simulink model "SpiderHalfCentre_SingleLeg"  (R2022b)
settings: Solver=ode4  StartTime=0.0  StopTime=30  FixedStep=1e-3  RelTol=1e-3
undefined symbols (not defined in the file): t1, t2, Vus0
libraries: vexv5lib x4, vexcommonlib x2, Vex_V5_Simulink_Expansion x2
settings Model: Creator=Serious Chimp  LastModifiedBy=Serious Chimp
settings SolverCC: EnableFixedStepZeroCrossing=on
settings OptimizationCC: EnhancedBackFolding=on  PassReuseOutputArgsAs=Individual arguments  ZeroExternalMemoryAtStartup=off  ZeroInternalMemoryAtStartup=off  MaxStackSize=64  OptimizeBlockOrder=speed  DifferentSizesBufferReuse=on  OptimizationCustomize=off  EfficientTunableParamExpr=on
settings DebuggingCC: ParameterTunabilityLossMsg=error
settings HardwareCC: ProdBitPerPointer=32  ProdBitPerSizeT=32  ProdBitPerPtrDiffT=32  ProdLargestAtomicInteger=Long  ProdLargestAtomicFloat=Double  ProdWordSize=32  ProdHWDeviceType=ARM Compatible->ARM Cortex  UseEmbeddedCoderFeatures=off
settings SFSimCC: MATLABDynamicMemAlloc=off
settings RTWCC: Description=Embedded Coder  SystemTargetFile=ert.tlc  HardwareBoard=VEX V5 Robot Brain  TLCOptions="-aInlineSetEventsForThisBaseRateFcn=TLC_FALSE -aSuppressMultiTaskScheduler=TLC_FALSE  -aRateBasedStepFcn=0"  TemplateMakefile=ert_default_tmf  Toolchain=GNU Tools for ARM Embedded Processors
settings CodeAppCC: ForceParamTrailComments=on  IgnoreCustomStorageClasses=off  OperatorAnnotations=on  SimulinkDataObjDesc=on  SFDataObjDesc=on  InsertBlockDesc=on
settings ERTTargetCC: SupportNonInlinedSFcns=on  ExtModeTransport=3  ExtModeStaticAlloc=on  ExtModeStaticAllocSize=2048  ExtModeMexFile=ext_xcp  ExtModeIntrfLevel=Level2 - Open

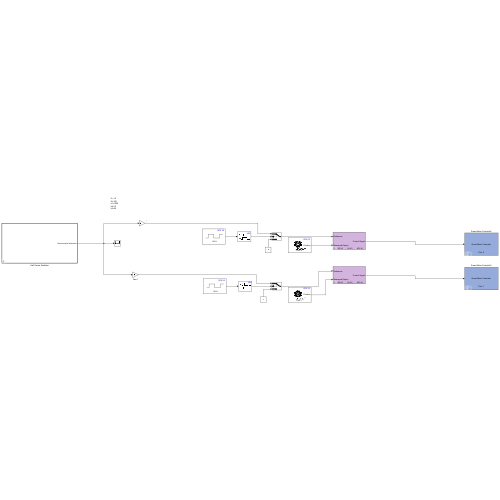
[thumbnail: Simulink's stored preview of the top-level diagram]
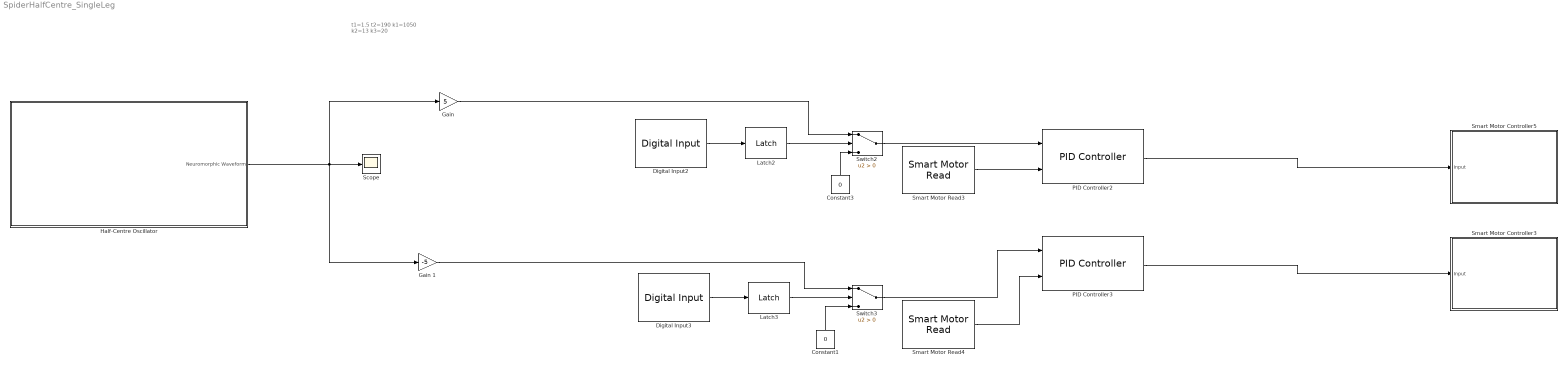
== system SpiderHalfCentre_SingleLeg ==
  note: t1=1.5
      | t2=190
      | k1=1050
      | k2=13
      | k3=20
  Constant1 : Constant  Value=0
  Constant3 : Constant  Value=0
  Digital Input2 : vexv5lib/Sensors/Digital Input  smartPort3wire=None  port=H  SampleTime=0.2
  Digital Input3 : vexv5lib/Sensors/Digital Input  smartPort3wire=None  port=H  SampleTime=0.2
  Gain : Gain  Gain=5
  Gain 1 : Gain  Gain=-5
  Half-Centre Oscillator : Subsystem  TreatAsAtomicUnit=on  mask{tau_s_A=t1, tau_us_A=t2, GB_A=-20, tau_s_B=t1, tau_us_B=t2, GB_B=-20, pain_threshold=2, pain_intensity=2, delay=0}
      mask prompts: tau_s_A "A - tau_s"; tau_us_A "A - tau_us"; GB_A "A - Inhibitory Synapse Threshold, GB_A"; tau_s_B "B - tau_s"; tau_us_B "B - tau_us"; GB_B "B - Inhibitory Synapse Threshold, GB_B"; pain_threshold "Range of Motion Position Threshold, pain_threshold"; pain_intensity "Range of Motion Intensity, pain_intensity"
  Latch2 : vexcommonlib/Latch  output0=off  BlockPlatform=vexv5
      settings: LibrarySourceBlock=vexv5lib/Utilities/Latch
  Latch3 : vexcommonlib/Latch  output0=off  BlockPlatform=vexv5
      settings: LibrarySourceBlock=vexv5lib/Utilities/Latch
  PID Controller2 : Vex_V5_Simulink_Expansion/Core Blocks/PID Controller  KP=k1  KI=k3  KD=k2  LimitOutput=off  limitHigh=0  limitLow=0  AntiWindupMode=none  kb=0
  PID Controller3 : Vex_V5_Simulink_Expansion/Core Blocks/PID Controller  KP=k1  KI=k3  KD=k2  LimitOutput=off  limitHigh=0  limitLow=0  AntiWindupMode=none  kb=0
  Scope : Scope
  Smart Motor Controller3 : Subsystem  AncestorBlock=Vex_V5_Simulink_Expansion/Core Blocks/Smart Motor Controller  mask(Smart Motor Controller){motorPort=1, OperationMode=Advanced Control, MotorBrakeMode=Coast}
      mask prompts: motorPort "Smart Port:"; OperationMode "Control Mode:"; MotorBrakeMode "Braking Mode:"
      mask help: Controls the Vex Smart Motor via the chosen method.
      mask TypeOptions motorPort: Advanced_SmartMotorWrite/motorPort
      mask TypeOptions OperationMode: Advanced_SmartMotorWrite/OperationMode
      mask TypeOptions MotorBrakeMode: Advanced_SmartMotorWrite/MotorBrakeMode
      mask DialogControl Container3 Prompt: Smart Motor Configuration
      mask Display:
      | %mode = get_param(gcb, 'control');
      | port = get_param(gcb, 'motorPort');
      | %text(0.3,0.45,[mode]);
      | 
      | text(0.5,0.5, 'Smart Motor Controller','HorizontalAlignment','center');
      | text(0.42,0.15, ['Port: ',port]);
  Smart Motor Controller5 : Subsystem  AncestorBlock=Vex_V5_Simulink_Expansion/Core Blocks/Smart Motor Controller  mask(Smart Motor Controller){motorPort=2, OperationMode=Advanced Control, MotorBrakeMode=Coast}
      mask prompts: motorPort "Smart Port:"; OperationMode "Control Mode:"; MotorBrakeMode "Braking Mode:"
      mask help: Controls the Vex Smart Motor via the chosen method.
      mask TypeOptions motorPort: Advanced_SmartMotorWrite/motorPort
      mask TypeOptions OperationMode: Advanced_SmartMotorWrite/OperationMode
      mask TypeOptions MotorBrakeMode: Advanced_SmartMotorWrite/MotorBrakeMode
      mask DialogControl Container3 Prompt: Smart Motor Configuration
      mask Display:
      | %mode = get_param(gcb, 'control');
      | port = get_param(gcb, 'motorPort');
      | %text(0.3,0.45,[mode]);
      | 
      | text(0.5,0.5, 'Smart Motor Controller','HorizontalAlignment','center');
      | text(0.42,0.15, ['Port: ',port]);
  Smart Motor Read3 : vexv5lib/Sensors/Smart Motor Read  motorPort=2  EncoderUnit=Degrees  resetOption=No reset  additionalOutput=off  SampleTime=0.01
  Smart Motor Read4 : vexv5lib/Sensors/Smart Motor Read  motorPort=1  EncoderUnit=Degrees  resetOption=No reset  additionalOutput=off  SampleTime=0.01
  Switch2 : Switch  Criteria=u2 > Threshold  SaturateOnIntegerOverflow=off  InputSameDT=off
  Switch3 : Switch  Criteria=u2 > Threshold  SaturateOnIntegerOverflow=off  InputSameDT=off
  wires:
  Smart Motor Read3/1 -> PID Controller2/2
  PID Controller2/1 -> Smart Motor Controller5/1(" Input")
  Gain 1/1 -> Switch3/1
  Digital Input2/1 -> Latch2/1
  Smart Motor Read4/1 -> PID Controller3/2
  Switch3/1 -> PID Controller3/1
  Constant3/1 -> Switch2/3
  Constant1/1 -> Switch3/3
  PID Controller3/1 -> Smart Motor Controller3/1(" Input")
  Gain/1 -> Switch2/1
  Latch3/1 -> Switch3/2
  Switch2/1 -> PID Controller2/1
  Digital Input3/1 -> Latch3/1
  Latch2/1 -> Switch2/2
  Half-Centre Oscillator/1(Neuromorphic Waveform) -> Scope/1, Gain/1, Gain 1/1

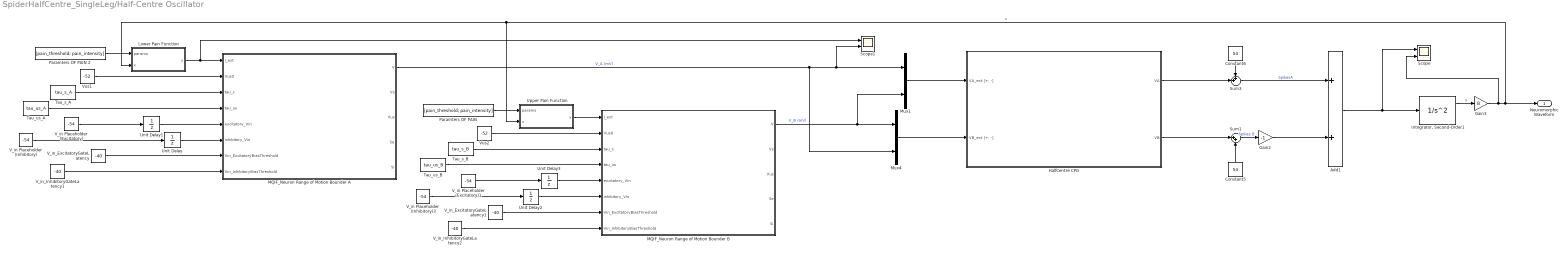
== system SpiderHalfCentre_SingleLeg/Half-Centre Oscillator ==
  Add1 : Sum
  Constant5 : Constant  Value=54
  Constant6 : Constant  Value=54
  Gain2 : Gain  Gain=-1
  Gain3 : Gain  Gain=8
  HalfCentre CPG : Subsystem  TreatAsAtomicUnit=on  mask{tau_s_A=t1, tau_us_A=t2, gSyn_excitatory_A=0.5, gSyn_inhibitory_A=0.5, tauSyn_excitatory_A=50, tauSyn_inhibitory_A=50, GB_A=-20, tau_s_B=t1, tau_us_B=t2, gSyn_excitatory_B=0.5, gSyn_inhibitory_B=0.5, tauSyn_excitatory_B=50, tauSyn_inhibitory_B=50, GB_B=-15, GB_excitatory=-40}
      mask prompts: tau_s_A "A - tau_s"; tau_us_A "A - tau_us"; gSyn_excitatory_A "A - Excitatory Synaptic Conductance, gSyn_excitatory"; gSyn_inhibitory_A "A - Inhibitory Synaptic Conductance, gSyn_inhibitory"; tauSyn_excitatory_A "A - Excitatory Synaptic Time Constant, tauSyn_excitatory"; tauSyn_inhibitory_A "A - Inhibitory Synaptic Time Constant, tauSyn_inhibitory"; GB_A "A - Inhibitory Synapse Threshold, GB_A"; tau_s_B "B - tau_s"; tau_us_B "B - tau_us"; gSyn_excitatory_B "B - Excitatory Synaptic Conductance, gSyn_excitatory"; gSyn_inhibitory_B "B - Inhibitory Synaptic Conductance, gSyn_inhibitory"; tauSyn_excitatory_B "B - Excitatory Synaptic Time Constant, tauSyn_excitatory"; tauSyn_inhibitory_B "B - Inhibitory Synaptic Time Constant, tauSyn_inhibitory"; GB_B "B - Inhibitory Synapse Threshold, GB_B"; GB_excitatory "Excitatory Gate Biases, GB_excitatory"
      mask Display: image('$imagefile'); % Use "Edit Image" on toolstrip to change.
  "Integrator, Second-Order1" : SecondOrderIntegrator
  Lower Pain Function : MATLAB Function  TreatAsAtomicUnit=on
  MQIF_Neuron Range of Motion Bounder A : Subsystem  TreatAsAtomicUnit=on  mask{V0=-52, Vs0=-50, V_threshold=20, V_reset=-45, Vs_reset=7.5, delta_Vus=1.7, g_f=1.0, g_s=0.5, g_us=0.015, C=0.82, Ve_syn=0, Vi_syn=-80, g_syn_excitatory=45, g_syn_inhibitory=45, tauSyn_excitatory=7, tauSyn_inhibitory=7, k=250}
      mask prompts: V0 "Equilibrium V0"; Vs0 "Equilibrium Vs0"; V_threshold "Threshold for Spike, V_thresh"; V_reset "After-spike Reset Votlage, V_r"; Vs_reset "After-spike Reset Vs, Vs_r"; delta_Vus "Vus After-spike Memory, delta_Vus"; g_f "I Conductance, g_f"; g_s "I_us Conductance, g_s"; g_us "I_us Conductance, g_us"; C "Capacitance, C"; Ve_syn "Equilibrium Inhibitory Synapse Voltage, Ve_syn"; Vi_syn "Equilibrium Inhibitory Synapse Voltage, Vi_syn"; g_syn_excitatory "Excitatory Synapse Conductance, g_syn_excitatory"; g_syn_inhibitory "Inhibitory Synapse Conductance, g_syn_inhibitory"; tauSyn_excitatory "Excitatory Synapse Time Constant, tauSyn_excitatory"; tauSyn_inhibitory "Inhibitory Synapse Time Constant, tauSyn_inhibitory"; k "Speed/Rate Constant, k"
      mask DialogControl NeuronStateVariables Prompt: Parameters
  MQIF_Neuron Range of Motion Bounder B : Subsystem  TreatAsAtomicUnit=on  mask{V0=-52, Vs0=-50, V_threshold=20, V_reset=-45, Vs_reset=7.5, delta_Vus=1.7, g_f=1.0, g_s=0.5, g_us=0.015, C=0.82, Ve_syn=0, Vi_syn=-80, g_syn_excitatory=45, g_syn_inhibitory=45, tauSyn_excitatory=7, tauSyn_inhibitory=7, k=250}
      mask prompts: V0 "Equilibrium V0"; Vs0 "Equilibrium Vs0"; V_threshold "Threshold for Spike, V_thresh"; V_reset "After-spike Reset Votlage, V_r"; Vs_reset "After-spike Reset Vs, Vs_r"; delta_Vus "Vus After-spike Memory, delta_Vus"; g_f "I Conductance, g_f"; g_s "I_us Conductance, g_s"; g_us "I_us Conductance, g_us"; C "Capacitance, C"; Ve_syn "Equilibrium Inhibitory Synapse Voltage, Ve_syn"; Vi_syn "Equilibrium Inhibitory Synapse Voltage, Vi_syn"; g_syn_excitatory "Excitatory Synapse Conductance, g_syn_excitatory"; g_syn_inhibitory "Inhibitory Synapse Conductance, g_syn_inhibitory"; tauSyn_excitatory "Excitatory Synapse Time Constant, tauSyn_excitatory"; tauSyn_inhibitory "Inhibitory Synapse Time Constant, tauSyn_inhibitory"; k "Speed/Rate Constant, k"
      mask DialogControl NeuronStateVariables Prompt: Parameters
  Mux1 : Mux  Inputs=2
  Mux4 : Mux  Inputs=2
  Paramters OF PAIN : Constant  Value=[pain_threshold; pain_intensity]
  Paramters OF PAIN 2 : Constant  Value=[pain_threshold; pain_intensity]
  Scope : Scope  NumInputPorts=2
  Scope1 : Scope  NumInputPorts=2
  Sum1 : Sum  Inputs=|++
  Sum3 : Sum  Inputs=++|
  Tau_s_A : Constant  Value=tau_s_A
  Tau_s_B : Constant  Value=tau_s_B
  Tau_us_A : Constant  Value=tau_us_A
  Tau_us_B : Constant  Value=tau_us_B
  Unit Delay{,1..3} (4 alike) : UnitDelay  InitialCondition=-54  SampleTime=-1  HasFrameUpgradeWarning=on
  Upper Pain Function : MATLAB Function  TreatAsAtomicUnit=on
  V_in Placeholder (Excitatory) : Constant  Value=-54
  V_in Placeholder (Excitatory)1 : Constant  Value=-54
  V_in Placeholder (Inhibitory) : Constant  Value=-54
  V_in Placeholder (Inhibitory)3 : Constant  Value=-54
  V_in_ExcitatoryGateLatency : Constant  Value=-40
  V_in_ExcitatoryGateLatency1 : Constant  Value=-40
  V_in_InhibitoryGateLatency1 : Constant  Value=-40
  V_in_InhibitoryGateLatency2 : Constant  Value=-40
  Vus1 : Constant  Value=-52
  Vus2 : Constant  Value=-52
  Neuromorphic Waveform : Outport
  wires:
  Constant5/1 -> Sum1/2
  MQIF_Neuron Range of Motion Bounder B/1(V) -> Mux1/2, Mux4/1  "V_B (mV)"
  V_in_ExcitatoryGateLatency/1 -> MQIF_Neuron Range of Motion Bounder A/7(Vin_ExcitatoryBiasThreshold)
  V_in Placeholder (Inhibitory)3/1 -> Unit Delay2/1
  Gain2/1 -> Add1/2
  V_in_InhibitoryGateLatency2/1 -> MQIF_Neuron Range of Motion Bounder B/8(Vin_InhibitoryBiasThreshold)
  Vus1/1 -> MQIF_Neuron Range of Motion Bounder A/2(Vus0)
  V_in Placeholder (Excitatory)/1 -> Unit Delay1/1
  Mux4/1 -> HalfCentre CPG/2(VB_ext [+; -])
  Unit Delay2/1 -> MQIF_Neuron Range of Motion Bounder B/6(inhibitory_Vin)
  Unit Delay/1 -> MQIF_Neuron Range of Motion Bounder A/6(inhibitory_Vin)
  Tau_s_B/1 -> MQIF_Neuron Range of Motion Bounder B/3(tau_s)
  Vus2/1 -> MQIF_Neuron Range of Motion Bounder B/2(Vus0)
  V_in Placeholder (Inhibitory)/1 -> Unit Delay/1
  "Integrator, Second-Order1"/1 -> Gain3/1  "x"
  V_in_ExcitatoryGateLatency1/1 -> MQIF_Neuron Range of Motion Bounder B/7(Vin_ExcitatoryBiasThreshold)
  Gain3/1 -> Scope/2, Neuromorphic Waveform/1, Upper Pain Function/2(x), Lower Pain Function/2(x)  "x"
  Sum3/1 -> Add1/1  "SpikesA"
  HalfCentre CPG/1(VA) -> Sum3/2
  V_in Placeholder (Excitatory)1/1 -> Unit Delay3/1
  Tau_us_A/1 -> MQIF_Neuron Range of Motion Bounder A/4(tau_us)
  Add1/1 -> Scope/1, "Integrator, Second-Order1"/1
  V_in_InhibitoryGateLatency1/1 -> MQIF_Neuron Range of Motion Bounder A/8(Vin_InhibitoryBiasThreshold)
  Unit Delay1/1 -> MQIF_Neuron Range of Motion Bounder A/5(excitatory_Vin)
  MQIF_Neuron Range of Motion Bounder A/1(V) -> Mux4/2, Scope1/2, Mux1/1  "V_A (mV)"
  Tau_s_A/1 -> MQIF_Neuron Range of Motion Bounder A/3(tau_s)
  Lower Pain Function/1(y) -> Scope1/1, MQIF_Neuron Range of Motion Bounder A/1(I_ext)
  Tau_us_B/1 -> MQIF_Neuron Range of Motion Bounder B/4(tau_us)
  Mux1/1 -> HalfCentre CPG/1(VA_ext [+; -])
  HalfCentre CPG/2(VB) -> Sum1/1
  Sum1/1 -> Gain2/1  "Spikes B"
  Unit Delay3/1 -> MQIF_Neuron Range of Motion Bounder B/5(excitatory_Vin)
  Constant6/1 -> Sum3/1
  Upper Pain Function/1(y) -> MQIF_Neuron Range of Motion Bounder B/1(I_ext)
  Paramters OF PAIN 2/1 -> Lower Pain Function/1(params)
  Paramters OF PAIN/1 -> Upper Pain Function/1(params)

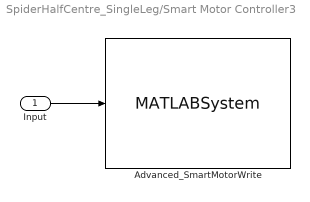
== system SpiderHalfCentre_SingleLeg/Smart Motor Controller3 ==
  " Input" : Inport
  Advanced_SmartMotorWrite : MATLABSystem  System=Advanced_SmartMotorWrite  motorPort=1  scaleFactor=36:1  MotorBrakeMode=Coast  OperationMode=Advanced Control
      mask Type: Advanced_SmartMotorWrite
      mask Display:
      | color('white');
      | plot([100,100,100,100]*1,[100,100,100,100]*1);
      | plot([100,100,100,100]*0,[100,100,100,100]*0);
      | color('black');
      | image(fullfile(codertarget.vexv5.internal.getSpPkgRootDir, 'resources', 'vex-v5-motor2.png'),'center');
      | patch([0.8, 0.8, 1, 1], [0.82857, 1, 1, 0.82857], [1, 1, 1]);
      | color('blue');
      | text(99, 92, 'VEX V5 ', 'horizontalAlignment', 'right');
      | color('black');
      | text(62,12,'Port: 1','horizontalAlignment','center');
      | 
      | port_label('Input',1,'Voltage(mV)');
  wires:
  " Input"/1 -> Advanced_SmartMotorWrite/1

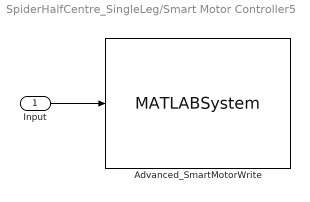
== system SpiderHalfCentre_SingleLeg/Smart Motor Controller5 ==
  " Input" : Inport
  Advanced_SmartMotorWrite : MATLABSystem  System=Advanced_SmartMotorWrite  motorPort=2  scaleFactor=36:1  MotorBrakeMode=Coast  OperationMode=Advanced Control
      mask Type: Advanced_SmartMotorWrite
      mask Display:
      | color('white');
      | plot([100,100,100,100]*1,[100,100,100,100]*1);
      | plot([100,100,100,100]*0,[100,100,100,100]*0);
      | color('black');
      | image(fullfile(codertarget.vexv5.internal.getSpPkgRootDir, 'resources', 'vex-v5-motor2.png'),'center');
      | patch([0.8, 0.8, 1, 1], [0.82857, 1, 1, 0.82857], [1, 1, 1]);
      | color('blue');
      | text(99, 92, 'VEX V5 ', 'horizontalAlignment', 'right');
      | color('black');
      | text(62,12,'Port: 2','horizontalAlignment','center');
      | 
      | port_label('Input',1,'Voltage(mV)');
  wires:
  " Input"/1 -> Advanced_SmartMotorWrite/1

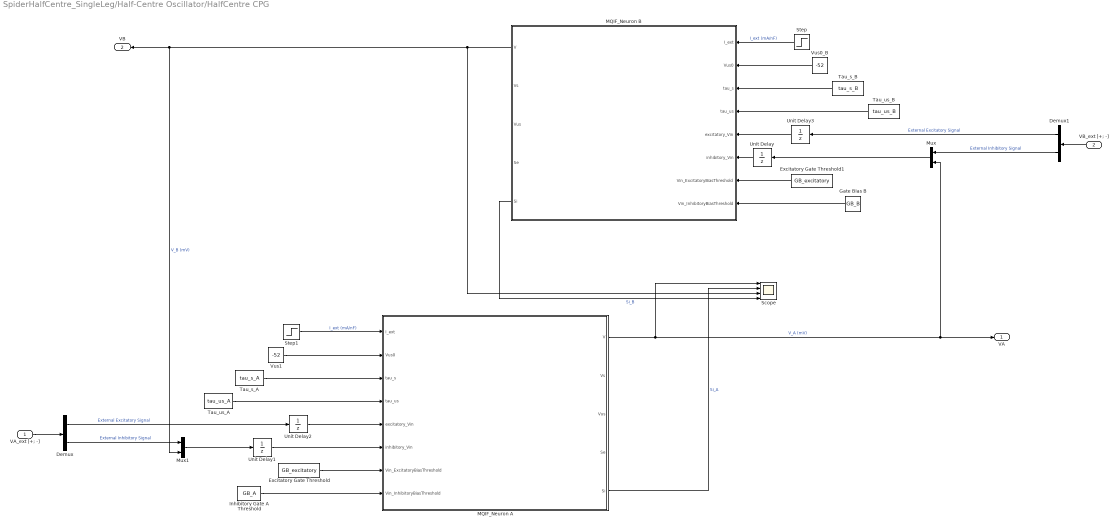
== system SpiderHalfCentre_SingleLeg/Half-Centre Oscillator/HalfCentre CPG ==
  VA_ext [+; -] : Inport
  VB_ext [+; -] : Inport  Port=2
  Demux : Demux  Outputs=2
  Demux1 : Demux  Outputs=2
  Excitatory Gate Threshold : Constant  Value=GB_excitatory
  Excitatory Gate Threshold1 : Constant  Value=GB_excitatory
  Gate BIas B : Constant  Value=GB_B
  Inhibitory Gate A Threshold : Constant  Value=GB_A
  MQIF_Neuron A : Subsystem  TreatAsAtomicUnit=on  mask{V0=-52, Vs0=-50, V_threshold=20, V_reset=-45, Vs_reset=7.5, delta_Vus=1.7, g_f=1.0, g_s=0.5, g_us=0.015, C=0.82, Ve_syn=0, Vi_syn=-90, g_syn_excitatory=gSyn_excitatory_A, g_syn_inhibitory=gSyn_inhibitory_A, tauSyn_excitatory=tauSyn_excitatory_A, tauSyn_inhibitory=tauSyn_inhibitory_A, k=250}
      mask prompts: V0 "Equilibrium V0"; Vs0 "Equilibrium Vs0"; V_threshold "Threshold for Spike, V_thresh"; V_reset "After-spike Reset Votlage, V_r"; Vs_reset "After-spike Reset Vs, Vs_r"; delta_Vus "Vus After-spike Memory, delta_Vus"; g_f "I Conductance, g_f"; g_s "I_us Conductance, g_s"; g_us "I_us Conductance, g_us"; C "Capacitance, C"; Ve_syn "Equilibrium Inhibitory Synapse Voltage, Ve_syn"; Vi_syn "Equilibrium Inhibitory Synapse Voltage, Vi_syn"; g_syn_excitatory "Excitatory Synapse Conductance, g_syn_excitatory"; g_syn_inhibitory "Inhibitory Synapse Conductance, g_syn_inhibitory"; tauSyn_excitatory "Excitatory Synapse Time Constant, tauSyn_excitatory"; tauSyn_inhibitory "Inhibitory Synapse Time Constant, tauSyn_inhibitory"; k "Speed/Rate Constant, k"
      mask DialogControl NeuronStateVariables Prompt: Parameters
  MQIF_Neuron B : Subsystem  TreatAsAtomicUnit=on  mask{V0=-52, Vs0=-50, V_threshold=20, V_reset=-45, Vs_reset=7.5, delta_Vus=1.7, g_f=1.0, g_s=0.5, g_us=0.015, C=0.82, Ve_syn=0, Vi_syn=-90, g_syn_excitatory=gSyn_excitatory_B, g_syn_inhibitory=gSyn_inhibitory_B, tauSyn_excitatory=tauSyn_excitatory_B, tauSyn_inhibitory=tauSyn_inhibitory_B, k=250}
      mask prompts: V0 "Equilibrium V0"; Vs0 "Equilibrium Vs0"; V_threshold "Threshold for Spike, V_thresh"; V_reset "After-spike Reset Votlage, V_r"; Vs_reset "After-spike Reset Vs, Vs_r"; delta_Vus "Vus After-spike Memory, delta_Vus"; g_f "I Conductance, g_f"; g_s "I_us Conductance, g_s"; g_us "I_us Conductance, g_us"; C "Capacitance, C"; Ve_syn "Equilibrium Inhibitory Synapse Voltage, Ve_syn"; Vi_syn "Equilibrium Inhibitory Synapse Voltage, Vi_syn"; g_syn_excitatory "Excitatory Synapse Conductance, g_syn_excitatory"; g_syn_inhibitory "Inhibitory Synapse Conductance, g_syn_inhibitory"; tauSyn_excitatory "Excitatory Synapse Time Constant, tauSyn_excitatory"; tauSyn_inhibitory "Inhibitory Synapse Time Constant, tauSyn_inhibitory"; k "Speed/Rate Constant, k"
      mask DialogControl NeuronStateVariables Prompt: Parameters
  Mux : Mux  Inputs=2
  Mux1 : Mux  Inputs=2
  Scope : Scope  NumInputPorts=4
  Step : Step  Time=delay  After=5  SampleTime=0
  Step1 : Step  Time=delay  After=5  SampleTime=0
  Tau_s_A : Constant  Value=tau_s_A
  Tau_s_B : Constant  Value=tau_s_B
  Tau_us_A : Constant  Value=tau_us_A
  Tau_us_B : Constant  Value=tau_us_B
  Unit Delay : UnitDelay  InitialCondition=[-54; -54]  SampleTime=-1  HasFrameUpgradeWarning=on
  Unit Delay1 : UnitDelay  InitialCondition=[-54; -54]  SampleTime=-1  HasFrameUpgradeWarning=on
  Unit Delay2 : UnitDelay  InitialCondition=-54  SampleTime=-1  HasFrameUpgradeWarning=on
  Unit Delay3 : UnitDelay  InitialCondition=-54  SampleTime=-1  HasFrameUpgradeWarning=on
  Vus0_B : Constant  Value=-52
  Vus1 : Constant  Value=-52
  VA : Outport
  VB : Outport  Port=2
  wires:
  Vus0_B/1 -> MQIF_Neuron B/2(Vus0)
  Unit Delay/1 -> MQIF_Neuron B/6(inhibitory_Vin)
  Inhibitory Gate A Threshold/1 -> MQIF_Neuron A/8(Vin_InhibitoryBiasThreshold)
  Tau_us_B/1 -> MQIF_Neuron B/4(tau_us)
  Vus1/1 -> MQIF_Neuron A/2(Vus0)
  Step1/1 -> MQIF_Neuron A/1(I_ext)  "I_ext (mA/nF)"
  Tau_s_A/1 -> MQIF_Neuron A/3(tau_s)
  Tau_s_B/1 -> MQIF_Neuron B/3(tau_s)
  Tau_us_A/1 -> MQIF_Neuron A/4(tau_us)
  Step/1 -> MQIF_Neuron B/1(I_ext)  "I_ext (mA/nF)"
  Unit Delay1/1 -> MQIF_Neuron A/6(inhibitory_Vin)
  Gate BIas B/1 -> MQIF_Neuron B/8(Vin_InhibitoryBiasThreshold)
  VB_ext [+; -]/1 -> Demux1/1
  Mux/1 -> Unit Delay/1
  Mux1/1 -> Unit Delay1/1
  VA_ext [+; -]/1 -> Demux/1
  Excitatory Gate Threshold/1 -> MQIF_Neuron A/7(Vin_ExcitatoryBiasThreshold)
  Demux/1 -> Unit Delay2/1  "External Excitatory Signal"
  MQIF_Neuron A/1(V) -> Scope/1, VA/1, Mux/2  "V_A (mV)"
  Unit Delay3/1 -> MQIF_Neuron B/5(excitatory_Vin)
  Demux/2 -> Mux1/1  "External Inhibitory Signal"
  Unit Delay2/1 -> MQIF_Neuron A/5(excitatory_Vin)
  Demux1/2 -> Mux/1  "External Inhibitory Signal"
  Demux1/1 -> Unit Delay3/1  "External Excitatory Signal"
  Excitatory Gate Threshold1/1 -> MQIF_Neuron B/7(Vin_ExcitatoryBiasThreshold)
  MQIF_Neuron B/1(V) -> Scope/3, VB/1, Mux1/2  "V_B (mV)"
  MQIF_Neuron A/5(Si) -> Scope/2  "Si_A"
  MQIF_Neuron B/5(Si) -> Scope/4  "Si_B"

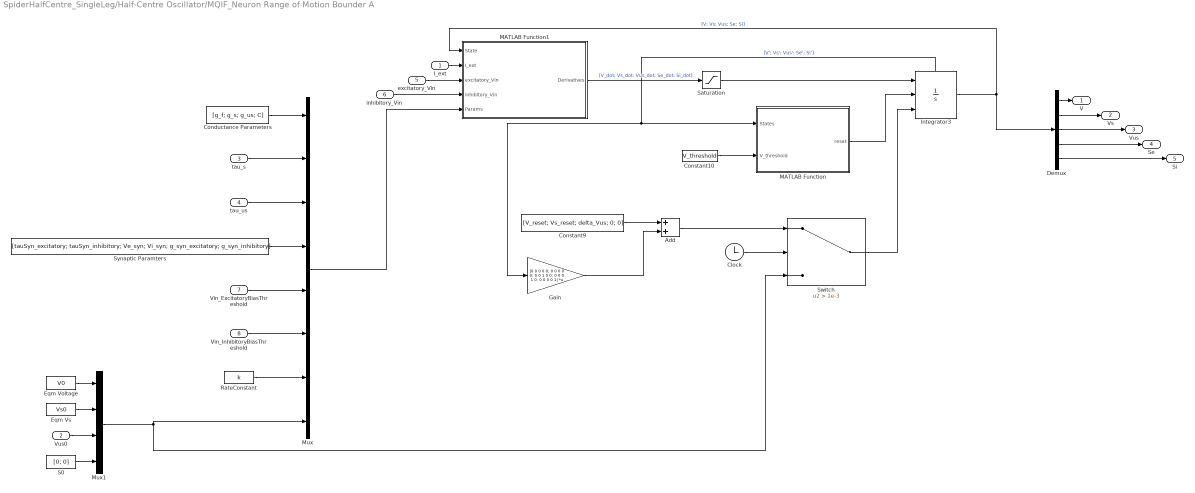
== system SpiderHalfCentre_SingleLeg/Half-Centre Oscillator/MQIF_Neuron Range of Motion Bounder A ==
  I_ext : Inport
  Vus0 : Inport  Port=2
  tau_s : Inport  Port=3
  tau_us : Inport  Port=4
  excitatory_Vin : Inport  Port=5
  inhibitory_Vin : Inport  Port=6
  Vin_ExcitatoryBiasThreshold : Inport  Port=7
  Vin_InhibitoryBiasThreshold : Inport  Port=8
  Add : Sum
  Clock : Clock
  Conductance Parameters : Constant  Value=[g_f; g_s; g_us; C]
  Constant10 : Constant  Value=V_threshold
  Constant9 : Constant  Value=[V_reset; Vs_reset; delta_Vus; 0; 0]
  Demux : Demux  Outputs=5
  Eqm Voltage : Constant  Value=V0
  Eqm Vs : Constant  Value=Vs0
  Gain : Gain  Gain=[0 0 0 0 0; 0 0 0 0 0; 0 0 1 0 0; 0 0 0 1 0; 0 0 0 0 1]  Multiplication=Matrix(K*u) (u vector)
  Integrator3 : Integrator  ExternalReset=rising  InitialConditionSource=external  InitialCondition=[V0 Vs0 Vus0]  ShowStatePort=on
  MATLAB Function : MATLAB Function  TreatAsAtomicUnit=on
  MATLAB Function1 : MATLAB Function  TreatAsAtomicUnit=on
  Mux : Mux  Inputs=8
  Mux1 : Mux
  RateConstant : Constant  Value=k
  S0 : Constant  Value=[0; 0]
  Saturation : Saturate  UpperLimit=1e4  LowerLimit=-1e4  LinearizeAsGain=off  ZeroCross=off
  Switch : Switch  Criteria=u2 > Threshold  Threshold=1e-3  SaturateOnIntegerOverflow=off  InputSameDT=off
  Synaptic Paramters : Constant  Value=[tauSyn_excitatory; tauSyn_inhibitory; Ve_syn; Vi_syn; g_syn_excitatory; g_syn_inhibitory]
  V : Outport
  Vs : Outport  Port=2
  Vus : Outport  Port=3
  Se : Outport  Port=4
  Si : Outport  Port=5
  wires:
  I_ext/1 -> MATLAB Function1/2(I_ext)
  Eqm Voltage/1 -> Mux1/1
  Vus0/1 -> Mux1/3
  Conductance Parameters/1 -> Mux/1
  tau_s/1 -> Mux/2
  tau_us/1 -> Mux/3
  Synaptic Paramters/1 -> Mux/4
  Mux/1 -> MATLAB Function1/5(Params)
  Constant10/1 -> MATLAB Function/2(V_threshold)
  Integrator3/1 -> MATLAB Function1/1(State), Demux/1  "[V; Vs; Vus; Se; Si]"
  Demux/1 -> V/1
  Demux/2 -> Vs/1
  Demux/3 -> Vus/1
  MATLAB Function/1(reset) -> Integrator3/2
  Clock/1 -> Switch/2
  Constant9/1 -> Add/1
  Switch/1 -> Integrator3/3
  Gain/1 -> Add/2
  MATLAB Function1/1(Derivatives) -> Saturation/1  "[V_dot; Vs_dot; Vus_dot; Se_dot; Si_dot]"
  Add/1 -> Switch/1
  Eqm Vs/1 -> Mux1/2
  inhibitory_Vin/1 -> MATLAB Function1/4(inhibitory_Vin)
  S0/1 -> Mux1/4
  Integrator3/State -> Gain/1, MATLAB Function/1(States)  "[V'; Vs'; Vus'; Se'; Si']"
  Demux/4 -> Se/1
  Vin_ExcitatoryBiasThreshold/1 -> Mux/5
  Saturation/1 -> Integrator3/1
  excitatory_Vin/1 -> MATLAB Function1/3(excitatory_Vin)
  Demux/5 -> Si/1
  RateConstant/1 -> Mux/7
  Mux1/1 -> Mux/8, Switch/3
  Vin_InhibitoryBiasThreshold/1 -> Mux/6

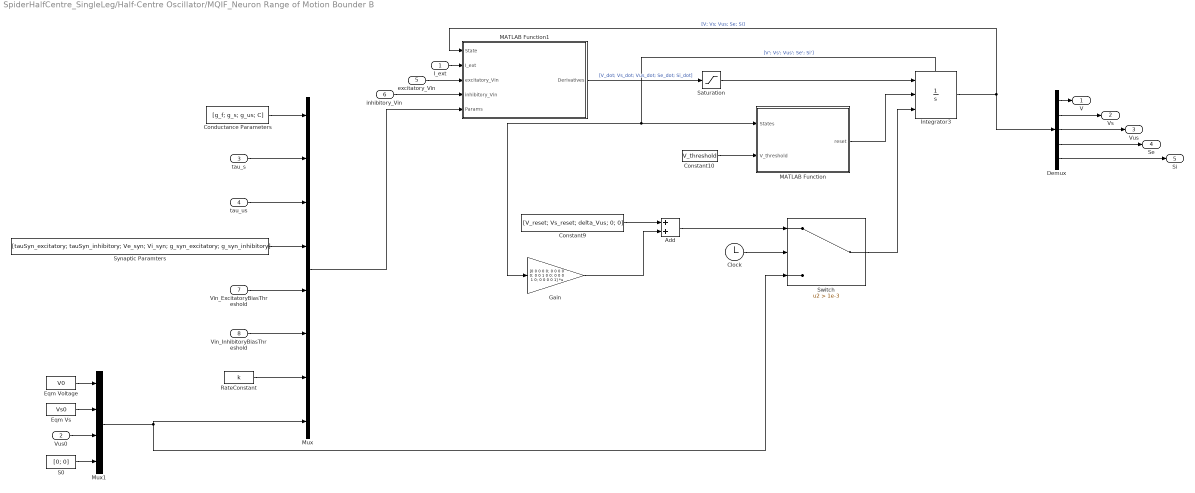
== system SpiderHalfCentre_SingleLeg/Half-Centre Oscillator/MQIF_Neuron Range of Motion Bounder B ==
  I_ext : Inport
  Vus0 : Inport  Port=2
  tau_s : Inport  Port=3
  tau_us : Inport  Port=4
  excitatory_Vin : Inport  Port=5
  inhibitory_Vin : Inport  Port=6
  Vin_ExcitatoryBiasThreshold : Inport  Port=7
  Vin_InhibitoryBiasThreshold : Inport  Port=8
  Add : Sum
  Clock : Clock
  Conductance Parameters : Constant  Value=[g_f; g_s; g_us; C]
  Constant10 : Constant  Value=V_threshold
  Constant9 : Constant  Value=[V_reset; Vs_reset; delta_Vus; 0; 0]
  Demux : Demux  Outputs=5
  Eqm Voltage : Constant  Value=V0
  Eqm Vs : Constant  Value=Vs0
  Gain : Gain  Gain=[0 0 0 0 0; 0 0 0 0 0; 0 0 1 0 0; 0 0 0 1 0; 0 0 0 0 1]  Multiplication=Matrix(K*u) (u vector)
  Integrator3 : Integrator  ExternalReset=rising  InitialConditionSource=external  InitialCondition=[V0 Vs0 Vus0]  ShowStatePort=on
  MATLAB Function : MATLAB Function  TreatAsAtomicUnit=on
  MATLAB Function1 : MATLAB Function  TreatAsAtomicUnit=on
  Mux : Mux  Inputs=8
  Mux1 : Mux
  RateConstant : Constant  Value=k
  S0 : Constant  Value=[0; 0]
  Saturation : Saturate  UpperLimit=1e4  LowerLimit=-1e4  LinearizeAsGain=off  ZeroCross=off
  Switch : Switch  Criteria=u2 > Threshold  Threshold=1e-3  SaturateOnIntegerOverflow=off  InputSameDT=off
  Synaptic Paramters : Constant  Value=[tauSyn_excitatory; tauSyn_inhibitory; Ve_syn; Vi_syn; g_syn_excitatory; g_syn_inhibitory]
  V : Outport
  Vs : Outport  Port=2
  Vus : Outport  Port=3
  Se : Outport  Port=4
  Si : Outport  Port=5
  wires:
  I_ext/1 -> MATLAB Function1/2(I_ext)
  Eqm Voltage/1 -> Mux1/1
  Vus0/1 -> Mux1/3
  Conductance Parameters/1 -> Mux/1
  tau_s/1 -> Mux/2
  tau_us/1 -> Mux/3
  Synaptic Paramters/1 -> Mux/4
  Mux/1 -> MATLAB Function1/5(Params)
  Constant10/1 -> MATLAB Function/2(V_threshold)
  Integrator3/1 -> MATLAB Function1/1(State), Demux/1  "[V; Vs; Vus; Se; Si]"
  Demux/1 -> V/1
  Demux/2 -> Vs/1
  Demux/3 -> Vus/1
  MATLAB Function/1(reset) -> Integrator3/2
  Clock/1 -> Switch/2
  Constant9/1 -> Add/1
  Switch/1 -> Integrator3/3
  Gain/1 -> Add/2
  MATLAB Function1/1(Derivatives) -> Saturation/1  "[V_dot; Vs_dot; Vus_dot; Se_dot; Si_dot]"
  Add/1 -> Switch/1
  Eqm Vs/1 -> Mux1/2
  inhibitory_Vin/1 -> MATLAB Function1/4(inhibitory_Vin)
  S0/1 -> Mux1/4
  Integrator3/State -> Gain/1, MATLAB Function/1(States)  "[V'; Vs'; Vus'; Se'; Si']"
  Demux/4 -> Se/1
  Vin_ExcitatoryBiasThreshold/1 -> Mux/5
  Saturation/1 -> Integrator3/1
  excitatory_Vin/1 -> MATLAB Function1/3(excitatory_Vin)
  Demux/5 -> Si/1
  RateConstant/1 -> Mux/7
  Mux1/1 -> Mux/8, Switch/3
  Vin_InhibitoryBiasThreshold/1 -> Mux/6

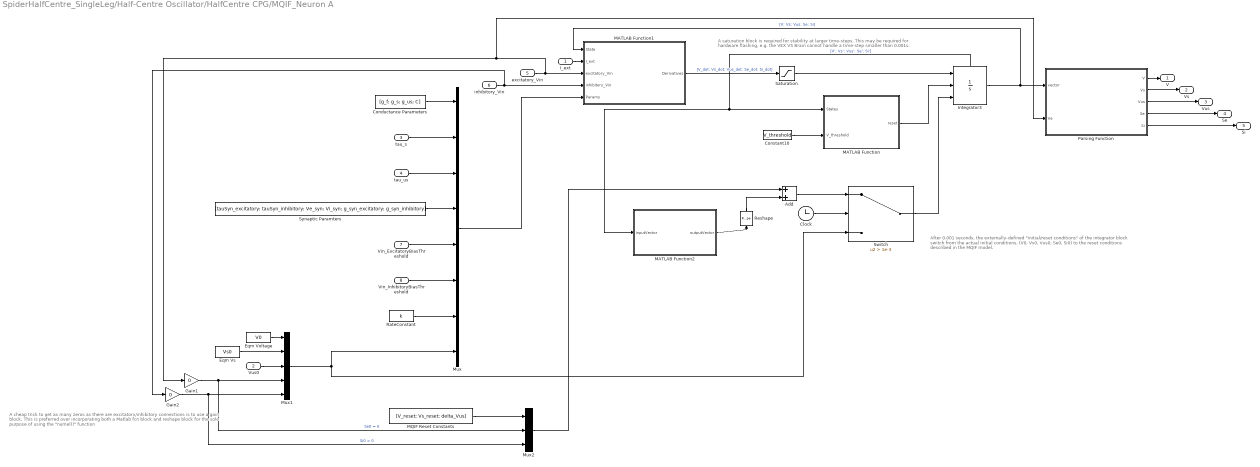
== system SpiderHalfCentre_SingleLeg/Half-Centre Oscillator/HalfCentre CPG/MQIF_Neuron A ==
  note: A saturation block is required for stability at larger time-steps. This may be required for hardware flashing, e.g. the VEX V5 Brain cannot handle a time-step smaller than 0.001s.
  note: After 0.001 seconds, the externally-defined "initial/reset conditions" of the integrator block switch from the actual initial conditions, (V0, Vs0, Vus0, Se0, Si0) to the reset conditions described in the MQIF model.
  note: A cheap trick to get as many zeros as there are excitatory/inhibitory connections
      | is to use a gain block. This is preferred over incorporating both a Matlab fcn block and reshape block for the sole purpose of using the "numel()" function
  I_ext : Inport
  Vus0 : Inport  Port=2
  tau_s : Inport  Port=3
  tau_us : Inport  Port=4
  excitatory_Vin : Inport  Port=5
  inhibitory_Vin : Inport  Port=6
  Vin_ExcitatoryBiasThreshold : Inport  Port=7
  Vin_InhibitoryBiasThreshold : Inport  Port=8
  Add : Sum
  Clock : Clock
  Conductance Parameters : Constant  Value=[g_f; g_s; g_us; C]
  Constant10 : Constant  Value=V_threshold
  Eqm Voltage : Constant  Value=V0
  Eqm Vs : Constant  Value=Vs0
  Gain1 : Gain  Gain=0
  Gain2 : Gain  Gain=0
  Integrator3 : Integrator  ExternalReset=rising  InitialConditionSource=external  InitialCondition=[V0 Vs0 Vus0]  ShowStatePort=on
  MATLAB Function : MATLAB Function  TreatAsAtomicUnit=on
  MATLAB Function1 : MATLAB Function  TreatAsAtomicUnit=on
  MATLAB Function2 : MATLAB Function  TreatAsAtomicUnit=on
  MQIF Reset Constants : Constant  Value=[V_reset; Vs_reset; delta_Vus]
  Mux : Mux  Inputs=8
  Mux1 : Mux  Inputs=5
  Mux2 : Mux  Inputs=3
  Parsing Function : MATLAB Function  TreatAsAtomicUnit=on
  RateConstant : Constant  Value=k
  Reshape : Reshape
  Saturation : Saturate  UpperLimit=1e4  LowerLimit=-1e4  LinearizeAsGain=off  ZeroCross=off
  Switch : Switch  Criteria=u2 > Threshold  Threshold=1e-3  SaturateOnIntegerOverflow=off  InputSameDT=off
  Synaptic Paramters : Constant  Value=[tauSyn_excitatory; tauSyn_inhibitory; Ve_syn; Vi_syn; g_syn_excitatory; g_syn_inhibitory]
  V : Outport
  Vs : Outport  Port=2
  Vus : Outport  Port=3
  Se : Outport  Port=4
  Si : Outport  Port=5
  wires:
  I_ext/1 -> MATLAB Function1/2(I_ext)
  Eqm Voltage/1 -> Mux1/1
  Vus0/1 -> Mux1/3
  Conductance Parameters/1 -> Mux/1
  tau_s/1 -> Mux/2
  tau_us/1 -> Mux/3
  Synaptic Paramters/1 -> Mux/4
  Mux/1 -> MATLAB Function1/5(Params)
  Constant10/1 -> MATLAB Function/2(V_threshold)
  Integrator3/1 -> MATLAB Function1/1(State), Parsing Function/1(vector)  "[V; Vs; Vus; Se; Si]"
  MATLAB Function/1(reset) -> Integrator3/2
  Clock/1 -> Switch/2
  MQIF Reset Constants/1 -> Mux2/1
  Switch/1 -> Integrator3/3
  MATLAB Function2/1(outputVector) -> Reshape/1
  MATLAB Function1/1(Derivatives) -> Saturation/1  "[V_dot; Vs_dot; Vus_dot; Se_dot; Si_dot]"
  Add/1 -> Switch/1
  Eqm Vs/1 -> Mux1/2
  inhibitory_Vin/1 -> Gain2/1, MATLAB Function1/4(inhibitory_Vin)
  Integrator3/State -> MATLAB Function2/1(inputVector), MATLAB Function/1(States)  "[V'; Vs'; Vus'; Se'; Si']"
  Vin_ExcitatoryBiasThreshold/1 -> Mux/5
  Saturation/1 -> Integrator3/1
  excitatory_Vin/1 -> Parsing Function/2(Ve), Gain1/1, MATLAB Function1/3(excitatory_Vin)
  RateConstant/1 -> Mux/7
  Mux1/1 -> Switch/3, Mux/8
  Vin_InhibitoryBiasThreshold/1 -> Mux/6
  Gain1/1 -> Mux1/4, Mux2/2  "Se0 = 0"
  Gain2/1 -> Mux2/3, Mux1/5  "Si0 = 0"
  Mux2/1 -> Add/1
  Reshape/1 -> Add/2
  Parsing Function/3(Vus) -> Vus/1
  Parsing Function/2(Vs) -> Vs/1
  Parsing Function/1(V) -> V/1
  Parsing Function/5(Si) -> Si/1
  Parsing Function/4(Se) -> Se/1

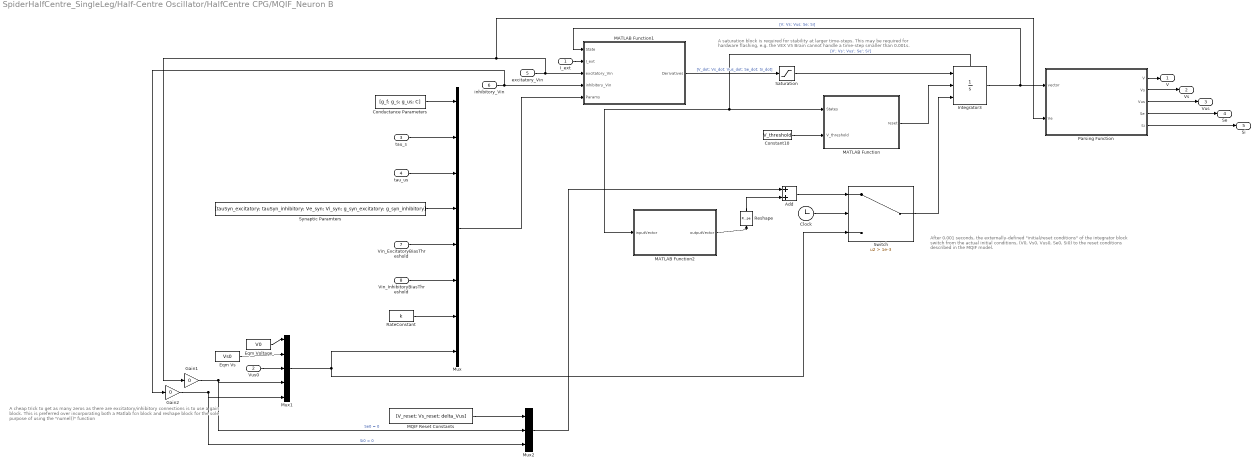
== system SpiderHalfCentre_SingleLeg/Half-Centre Oscillator/HalfCentre CPG/MQIF_Neuron B ==
  note: A saturation block is required for stability at larger time-steps. This may be required for hardware flashing, e.g. the VEX V5 Brain cannot handle a time-step smaller than 0.001s.
  note: After 0.001 seconds, the externally-defined "initial/reset conditions" of the integrator block switch from the actual initial conditions, (V0, Vs0, Vus0, Se0, Si0) to the reset conditions described in the MQIF model.
  note: A cheap trick to get as many zeros as there are excitatory/inhibitory connections
      | is to use a gain block. This is preferred over incorporating both a Matlab fcn block and reshape block for the sole purpose of using the "numel()" function
  I_ext : Inport
  Vus0 : Inport  Port=2
  tau_s : Inport  Port=3
  tau_us : Inport  Port=4
  excitatory_Vin : Inport  Port=5
  inhibitory_Vin : Inport  Port=6
  Vin_ExcitatoryBiasThreshold : Inport  Port=7
  Vin_InhibitoryBiasThreshold : Inport  Port=8
  Add : Sum
  Clock : Clock
  Conductance Parameters : Constant  Value=[g_f; g_s; g_us; C]
  Constant10 : Constant  Value=V_threshold
  Eqm Voltage : Constant  Value=V0
  Eqm Vs : Constant  Value=Vs0
  Gain1 : Gain  Gain=0
  Gain2 : Gain  Gain=0
  Integrator3 : Integrator  ExternalReset=rising  InitialConditionSource=external  InitialCondition=[V0 Vs0 Vus0]  ShowStatePort=on
  MATLAB Function : MATLAB Function  TreatAsAtomicUnit=on
  MATLAB Function1 : MATLAB Function  TreatAsAtomicUnit=on
  MATLAB Function2 : MATLAB Function  TreatAsAtomicUnit=on
  MQIF Reset Constants : Constant  Value=[V_reset; Vs_reset; delta_Vus]
  Mux : Mux  Inputs=8
  Mux1 : Mux  Inputs=5
  Mux2 : Mux  Inputs=3
  Parsing Function : MATLAB Function  TreatAsAtomicUnit=on
  RateConstant : Constant  Value=k
  Reshape : Reshape
  Saturation : Saturate  UpperLimit=1e4  LowerLimit=-1e4  LinearizeAsGain=off  ZeroCross=off
  Switch : Switch  Criteria=u2 > Threshold  Threshold=1e-3  SaturateOnIntegerOverflow=off  InputSameDT=off
  Synaptic Paramters : Constant  Value=[tauSyn_excitatory; tauSyn_inhibitory; Ve_syn; Vi_syn; g_syn_excitatory; g_syn_inhibitory]
  V : Outport
  Vs : Outport  Port=2
  Vus : Outport  Port=3
  Se : Outport  Port=4
  Si : Outport  Port=5
  wires:
  I_ext/1 -> MATLAB Function1/2(I_ext)
  Eqm Voltage/1 -> Mux1/1
  Vus0/1 -> Mux1/3
  Conductance Parameters/1 -> Mux/1
  tau_s/1 -> Mux/2
  tau_us/1 -> Mux/3
  Synaptic Paramters/1 -> Mux/4
  Mux/1 -> MATLAB Function1/5(Params)
  Constant10/1 -> MATLAB Function/2(V_threshold)
  Integrator3/1 -> MATLAB Function1/1(State), Parsing Function/1(vector)  "[V; Vs; Vus; Se; Si]"
  MATLAB Function/1(reset) -> Integrator3/2
  Clock/1 -> Switch/2
  MQIF Reset Constants/1 -> Mux2/1
  Switch/1 -> Integrator3/3
  MATLAB Function2/1(outputVector) -> Reshape/1
  MATLAB Function1/1(Derivatives) -> Saturation/1  "[V_dot; Vs_dot; Vus_dot; Se_dot; Si_dot]"
  Add/1 -> Switch/1
  Eqm Vs/1 -> Mux1/2
  inhibitory_Vin/1 -> Gain2/1, MATLAB Function1/4(inhibitory_Vin)
  Integrator3/State -> MATLAB Function2/1(inputVector), MATLAB Function/1(States)  "[V'; Vs'; Vus'; Se'; Si']"
  Vin_ExcitatoryBiasThreshold/1 -> Mux/5
  Saturation/1 -> Integrator3/1
  excitatory_Vin/1 -> Parsing Function/2(Ve), Gain1/1, MATLAB Function1/3(excitatory_Vin)
  RateConstant/1 -> Mux/7
  Mux1/1 -> Mux/8, Switch/3
  Vin_InhibitoryBiasThreshold/1 -> Mux/6
  Gain1/1 -> Mux1/4, Mux2/2  "Se0 = 0"
  Gain2/1 -> Mux2/3, Mux1/5  "Si0 = 0"
  Mux2/1 -> Add/1
  Reshape/1 -> Add/2
  Parsing Function/3(Vus) -> Vus/1
  Parsing Function/2(Vs) -> Vs/1
  Parsing Function/1(V) -> V/1
  Parsing Function/5(Si) -> Si/1
  Parsing Function/4(Se) -> Se/1

== matlab function SpiderHalfCentre_SingleLeg/Half-Centre Oscillator/MQIF_Neuron Range of Motion Bounder B/MATLAB Function ==
  data: States input; reset output; V_threshold input
function reset = ResetTrigger(States, V_threshold)

V = States(1);

reset = (V > V_threshold);

end

== matlab function SpiderHalfCentre_SingleLeg/Half-Centre Oscillator/MQIF_Neuron Range of Motion Bounder B/MATLAB Function1 ==
  data: State input; Derivatives output; I_ext input; excitatory_Vin input; inhibitory_Vin input; Params input
function Derivatives = ODE(State, I_ext, excitatory_Vin, inhibitory_Vin, Params)
    V = State(1);
    Vs = State(2);
    Vus = State(3);
    Se = State(4);
    Si = State(5);

    g_f = Params(1);
    g_s = Params(2);
    g_us = Params(3);
    C = Params(4);
    tau_s = Params(5);
    tau_us = Params(6);
    tau_syn_E = Params(7);
    tau_syn_I = Params(8);
    Ve_syn = Params(9);
    Vi_syn = Params(10);
    g_syn_E = Params(11);
    g_syn_I = Params(12);
    Vin_gate_E = Params(13);
    Vin_gate_I = Params(14);
    k = Params(15);
    V0 = Params(16);
    Vs0 = Params(17);
    Vus0 = Params(18);
  
    sigmoid_Ve = 1/(1+exp(-(40*(sum(excitatory_Vin)-Vin_gate_E))));
    sigmoid_Vi = 1/(1+exp(-(40*(sum(inhibitory_Vin)-Vin_gate_I))));
    
    V_dot = k*(((I_ext + g_f*((V-V0)^2) - g_s*((Vs-Vs0)^2) - g_us*((Vus-Vus0)^2) + g_syn_E*Se*(Ve_syn-V) +g_syn_I*Si*(Vi_syn-V)) / C));
    Vs_dot = k*((V - Vs) / tau_s);
    Vus_dot = k*((V - Vus) / tau_us);
    Se_dot = k*((sigmoid_Ve - Se)/tau_syn_E);
    Si_dot = k*((sigmoid_Vi - Si)/tau_syn_I);

    Derivatives = [V_dot; Vs_dot; Vus_dot; Se_dot; Si_dot];
end

== matlab function SpiderHalfCentre_SingleLeg/Half-Centre Oscillator/Upper Pain Function ==
  data: params input; x input; y output
function y = UpperRangeofMotion(params, x)
    c = params(1);
    u=params(2);
  
    y = 50/(1+exp(-u*(x-c)));
end

== matlab function SpiderHalfCentre_SingleLeg/Half-Centre Oscillator/HalfCentre CPG/MQIF_Neuron B/MATLAB Function1 ==
  data: State input; Derivatives output; I_ext input; excitatory_Vin input; inhibitory_Vin input; Params input
% This fcn implements the MQIF dynamics as ordinary differential equations.

function Derivatives = ODE(State, I_ext, excitatory_Vin, inhibitory_Vin, Params)
    % Parse through states
    V = State(1);
    Vs = State(2);
    Vus = State(3);
    Se = State(4:numel(excitatory_Vin)+3);
    Si = State(numel(excitatory_Vin)+4:end);

    % Parse through parameters
    g_f = Params(1);
    g_s = Params(2);
    g_us = Params(3);
    C = Params(4);
    tau_s = Params(5);
    tau_us = Params(6);
    tau_syn_E = Params(7);
    tau_syn_I = Params(8);
    Ve_syn = Params(9);
    Vi_syn = Params(10);
    g_syn_E = Params(11);
    g_syn_I = Params(12);
    Vin_gate_E = Params(13);
    Vin_gate_I = Params(14);
    k = Params(15);
    V0 = Params(16);
    Vs0 = Params(17);
    Vus0 = Params(18);

    % Non-linear function to control synaptic gating
    sigmoid_Ve = 1./(1+exp(-(40*(excitatory_Vin-Vin_gate_E))));
    sigmoid_Vi = 1./(1+exp(-(40*(inhibitory_Vin-Vin_gate_I))));

    % Excitatory and inhibitory currents
    I_excitatory = g_syn_E*Se*(Ve_syn-V);
    I_inhibitory = g_syn_I*Si*(Vi_syn-V);

    % ODE's that will be solved by the integrator block following this fcn
    V_dot = k*(((I_ext + g_f*((V-V0)^2) - g_s*((Vs-Vs0)^2) - g_us*((Vus-Vus0)^2) + sum(I_excitatory) + sum(I_inhibitory)) / C));
    Vs_dot = k*((V - Vs) / tau_s);
    Vus_dot = k*((V - Vus) / tau_us);
    Se_dot = k*((sigmoid_Ve - Se)/tau_syn_E);
    Si_dot = k*((sigmoid_Vi - Si)/tau_syn_I);

    Derivatives = [V_dot; Vs_dot; Vus_dot; Se_dot; Si_dot];
end

== matlab function SpiderHalfCentre_SingleLeg/Half-Centre Oscillator/Lower Pain Function ==
  data: params input; x input; y output
function y =  LowerRangeofMotion(params, x)
    c = params(1);
    u=params(2);
    
    y = 50/(1+exp(-u*(-x-c)));
end

== matlab function SpiderHalfCentre_SingleLeg/Half-Centre Oscillator/HalfCentre CPG/MQIF_Neuron B/MATLAB Function ==
  data: States input; reset output; V_threshold input
% This fcn triggers the reset of the following integrator block. When membrane
% potential rises above V_threshold, an action potential has been fired, 
% as specified for integrate-and-fire neuron behavior.

function reset = ResetTrigger(States, V_threshold)

V = States(1);

reset = (V > V_threshold);

end

== matlab function SpiderHalfCentre_SingleLeg/Half-Centre Oscillator/HalfCentre CPG/MQIF_Neuron A/MATLAB Function ==
  data: States input; reset output; V_threshold input
% This fcn triggers the reset of the following integrator block. When membrane
% potential rises above V_threshold, an action potential has been fired, 
% as specified for integrate-and-fire neuron behavior.

function reset = ResetTrigger(States, V_threshold)

V = States(1);

reset = (V > V_threshold);

end

== matlab function SpiderHalfCentre_SingleLeg/Half-Centre Oscillator/HalfCentre CPG/MQIF_Neuron A/MATLAB Function1 ==
  data: State input; Derivatives output; I_ext input; excitatory_Vin input; inhibitory_Vin input; Params input
% This fcn implements the MQIF dynamics as ordinary differential equations.

function Derivatives = ODE(State, I_ext, excitatory_Vin, inhibitory_Vin, Params)
    % Parse through states
    V = State(1);
    Vs = State(2);
    Vus = State(3);
    Se = State(4:numel(excitatory_Vin)+3);
    Si = State(numel(excitatory_Vin)+4:end);

    % Parse through parameters
    g_f = Params(1);
    g_s = Params(2);
    g_us = Params(3);
    C = Params(4);
    tau_s = Params(5);
    tau_us = Params(6);
    tau_syn_E = Params(7);
    tau_syn_I = Params(8);
    Ve_syn = Params(9);
    Vi_syn = Params(10);
    g_syn_E = Params(11);
    g_syn_I = Params(12);
    Vin_gate_E = Params(13);
    Vin_gate_I = Params(14);
    k = Params(15);
    V0 = Params(16);
    Vs0 = Params(17);
    Vus0 = Params(18);

    % Non-linear function to control synaptic gating
    sigmoid_Ve = 1./(1+exp(-(40*(excitatory_Vin-Vin_gate_E))));
    sigmoid_Vi = 1./(1+exp(-(40*(inhibitory_Vin-Vin_gate_I))));

    % Excitatory and inhibitory currents
    I_excitatory = g_syn_E*Se*(Ve_syn-V);
    I_inhibitory = g_syn_I*Si*(Vi_syn-V);

    % ODE's that will be solved by the integrator block following this fcn
    V_dot = k*(((I_ext + g_f*((V-V0)^2) - g_s*((Vs-Vs0)^2) - g_us*((Vus-Vus0)^2) + sum(I_excitatory) + sum(I_inhibitory)) / C));
    Vs_dot = k*((V - Vs) / tau_s);
    Vus_dot = k*((V - Vus) / tau_us);
    Se_dot = k*((sigmoid_Ve - Se)/tau_syn_E);
    Si_dot = k*((sigmoid_Vi - Si)/tau_syn_I);

    Derivatives = [V_dot; Vs_dot; Vus_dot; Se_dot; Si_dot];
end

== matlab function SpiderHalfCentre_SingleLeg/Half-Centre Oscillator/HalfCentre CPG/MQIF_Neuron A/MATLAB Function2 ==
  data: inputVector input; outputVector output
% This function is required to make sure that the MQIF neuron is input
% agnostic, (can handle any number of excitatory/inhibitory connections).
% 
% We require a matrix that can extract Vus (scalar), Se and Si (vectors of
% arbitrary length), and ignore the other values. This is because these
% values are "remembered" after each action potential and are required in
% the subsequent resetting of states.

function outputVector = generalisedMatrix(inputVector)
    % Get the size of the input vector
    n = length(inputVector);

    % Create a square matrix of zeros
    Matrix = zeros(n);

    % Set the (3, 3) element to 1
    Matrix(3, 3) = 1;

    % Set the values for every row i, starting from the fourth row
    for i = 4:n
        Matrix(i, i) = 1;
    end

    outputVector = Matrix*inputVector;
end

== matlab function SpiderHalfCentre_SingleLeg/Half-Centre Oscillator/HalfCentre CPG/MQIF_Neuron A/Parsing Function ==
  data: vector input; V output; Vs output; Vus output; Ve input; Se output; Si output
% This fcn parses through the vectorised input signal, to output the
% various states through the enclosing mask's outports. It is designed to
% be input agnostic, (i.e. the neuron can handle any number of excitatory/inhibitory
% connections, and it outputs Se and Si as vectorised signals).

function [V,Vs,Vus,Se,Si] = InputAgnosticDemux(vector, Ve)
    V = vector(1);
    Vs = vector(2);
    Vus = vector(3);
    Se = vector(4:numel(Ve)+3);
    Si = vector(numel(Ve)+4:end);
end

== matlab function SpiderHalfCentre_SingleLeg/Half-Centre Oscillator/MQIF_Neuron Range of Motion Bounder A/MATLAB Function ==
  data: States input; reset output; V_threshold input
function reset = ResetTrigger(States, V_threshold)

V = States(1);

reset = (V > V_threshold);

end

== matlab function SpiderHalfCentre_SingleLeg/Half-Centre Oscillator/MQIF_Neuron Range of Motion Bounder A/MATLAB Function1 ==
  data: State input; Derivatives output; I_ext input; excitatory_Vin input; inhibitory_Vin input; Params input
function Derivatives = ODE(State, I_ext, excitatory_Vin, inhibitory_Vin, Params)
    V = State(1);
    Vs = State(2);
    Vus = State(3);
    Se = State(4);
    Si = State(5);

    g_f = Params(1);
    g_s = Params(2);
    g_us = Params(3);
    C = Params(4);
    tau_s = Params(5);
    tau_us = Params(6);
    tau_syn_E = Params(7);
    tau_syn_I = Params(8);
    Ve_syn = Params(9);
    Vi_syn = Params(10);
    g_syn_E = Params(11);
    g_syn_I = Params(12);
    Vin_gate_E = Params(13);
    Vin_gate_I = Params(14);
    k = Params(15);
    V0 = Params(16);
    Vs0 = Params(17);
    Vus0 = Params(18);
  
    sigmoid_Ve = 1/(1+exp(-(40*(sum(excitatory_Vin)-Vin_gate_E))));
    sigmoid_Vi = 1/(1+exp(-(40*(sum(inhibitory_Vin)-Vin_gate_I))));
    
    V_dot = k*(((I_ext + g_f*((V-V0)^2) - g_s*((Vs-Vs0)^2) - g_us*((Vus-Vus0)^2) + g_syn_E*Se*(Ve_syn-V) +g_syn_I*Si*(Vi_syn-V)) / C));
    Vs_dot = k*((V - Vs) / tau_s);
    Vus_dot = k*((V - Vus) / tau_us);
    Se_dot = k*((sigmoid_Ve - Se)/tau_syn_E);
    Si_dot = k*((sigmoid_Vi - Si)/tau_syn_I);

    Derivatives = [V_dot; Vs_dot; Vus_dot; Se_dot; Si_dot];
end

== matlab function SpiderHalfCentre_SingleLeg/Half-Centre Oscillator/HalfCentre CPG/MQIF_Neuron B/MATLAB Function2 ==
  data: inputVector input; outputVector output
% This function is required to make sure that the MQIF neuron is input
% agnostic, (can handle any number of excitatory/inhibitory connections).
% 
% We require a matrix that can extract Vus (scalar), Se and Si (vectors of
% arbitrary length), and ignore the other values. This is because these
% values are "remembered" after each action potential and are required in
% the subsequent resetting of states.

function outputVector = generalisedMatrix(inputVector)
    % Get the size of the input vector
    n = length(inputVector);

    % Create a square matrix of zeros
    Matrix = zeros(n);

    % Set the (3, 3) element to 1
    Matrix(3, 3) = 1;

    % Set the values for every row i, starting from the fourth row
    for i = 4:n
        Matrix(i, i) = 1;
    end

    outputVector = Matrix*inputVector;
end

== matlab function SpiderHalfCentre_SingleLeg/Half-Centre Oscillator/HalfCentre CPG/MQIF_Neuron B/Parsing Function ==
  data: vector input; V output; Vs output; Vus output; Ve input; Se output; Si output
% This fcn parses through the vectorised input signal, to output the
% various states through the enclosing mask's outports. It is designed to
% be input agnostic, (i.e. the neuron can handle any number of excitatory/inhibitory
% connections, and it outputs Se and Si as vectorised signals).

function [V,Vs,Vus,Se,Si] = InputAgnosticDemux(vector, Ve)
    V = vector(1);
    Vs = vector(2);
    Vus = vector(3);
    Se = vector(4:numel(Ve)+3);
    Si = vector(numel(Ve)+4:end);
end
